simulink model "FTVsWBD_SingleSupportRightLeg"  (R2014a)
settings: Solver=ode45  StartTime=0.0  StopTime=5  RelTol=1e-3
libraries: WBCLibrary x3
settings Model: Creator=jorhabib  LastModifiedBy=jorhabib

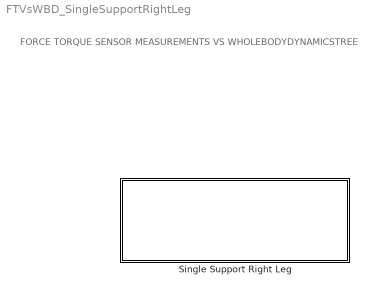
== system FTVsWBD_SingleSupportRightLeg ==
  note: FORCE TORQUE SENSOR MEASUREMENTS
      |                                     VS
      |             WHOLEBODYDYNAMICSTREE
  Single Support Right Leg : Subsystem  mask{robotName='iCubGenova01', localName='simulink', Ts=0.010}
      mask prompts: robotName "Robot Name"; localName "Local Name"; Ts "Simulation Period"

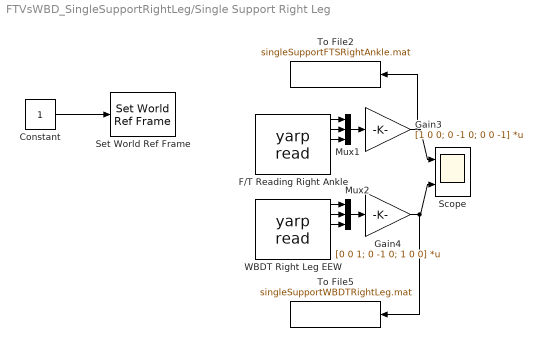
== system FTVsWBD_SingleSupportRightLeg/Single Support Right Leg ==
  Constant : Constant  OutDataTypeStr=int8  SampleTime=Ts
  F/T Reading Right Ankle : WBCLibrary/Utilities/yarp read  from=['/icub' '/right_foot/analog:o']  to='...'  num=6
  Gain3 : Gain  Gain=[1 0 0; 0 -1 0; 0 0 -1]  Multiplication=Matrix(K*u)  SampleTime=Ts
  Gain4 : Gain  Gain=[0 0 1; 0 -1 0; 1 0 0]  Multiplication=Matrix(K*u)  SampleTime=Ts
  Mux1 : Mux  Inputs=3
  Mux2 : Mux  Inputs=3
  Scope : Scope  NumInputPorts=2
      settings: ShowLegends=on  YMin=-20~-25  YMax=180~175
  Set World Ref Frame : WBCLibrary/wholeBodyModel/Set World Ref Frame  robotName=robotName  localName=localName
  To File2 : ToFile  Filename=singleSupportFTSRightAnkle.mat  MatrixName=singleSupportFTSRightAnkle  SaveFormat=Timeseries  SampleTime=Ts
  To File5 : ToFile  Filename=singleSupportWBDTRightLeg.mat  MatrixName=singleSupportWBDTRightLeg  SaveFormat=Timeseries  SampleTime=Ts
  WBDT Right Leg EEW : WBCLibrary/Utilities/yarp read  from=['/wholeBodyDynamicsTree' '/right_leg/endEffectorWrench:o']  to='...'  num=6
  wires:
  Constant/1 -> Set World Ref Frame/1
  WBDT Right Leg EEW/2 -> Mux2/2
  WBDT Right Leg EEW/1 -> Mux2/1
  WBDT Right Leg EEW/3 -> Mux2/3
  Gain4/1 -> To File5/1, Scope/2
  Gain3/1 -> To File2/1, Scope/1
  F/T Reading Right Ankle/1 -> Mux1/1
  F/T Reading Right Ankle/2 -> Mux1/2
  F/T Reading Right Ankle/3 -> Mux1/3
  Mux1/1 -> Gain3/1
  Mux2/1 -> Gain4/1
